simulink model "robot_capteur_etu"  (R2022a)
settings: Solver=VariableStepAuto  StartTime=0.0  StopTime=10.0  RelTol=1e-3
values from neighbouring files (symbols this model uses):
  K = -place(A,B,[-136.4009, -2.6408, -3.5890, -5.9800])    [matrices.m]    (also in simu_robot_etu.m = [0.6700 19.9055 1.0747  1.9614])
  ue = 0    [simu_robot_etu.m]
  x0 = [0 pi/10 0 0]    [simu_robot_etu.m]
  xe = [0 0 0 0]'    [simu_robot_etu.m]
settings Model: Creator=melallem  LastModifiedBy=elgue
settings DebuggingCC: UnconnectedInputMsg=warning  UnconnectedOutputMsg=warning  UnconnectedLineMsg=warning
settings RTWCC: DLArmComputeVersion=19.05

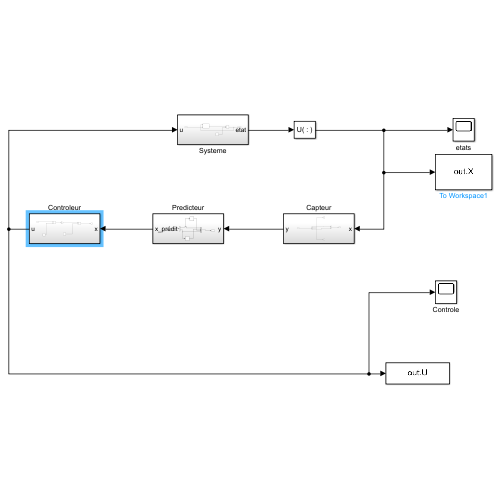
[thumbnail: Simulink's stored preview of the top-level diagram]
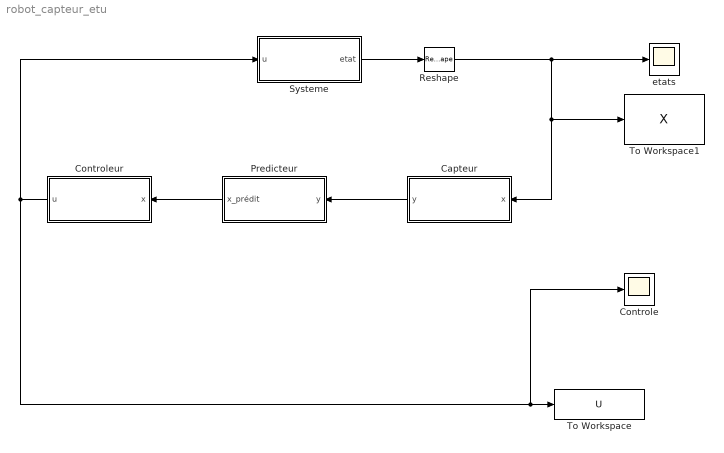
== system robot_capteur_etu ==
  Capteur : Subsystem
  Controle : Scope
  Controleur : Subsystem
  Predicteur : Subsystem
  Reshape : Reshape
  Systeme : Subsystem
  To Workspace : ToWorkspace  VariableName=U  SaveFormat=Timeseries  SampleTime=-1
  To Workspace1 : ToWorkspace  VariableName=X  SaveFormat=Timeseries  SampleTime=-1
  etats : Scope
  wires:
  Predicteur/1(x_prédit) -> Controleur/1(x)
  Capteur/1(y) -> Predicteur/1(y)
  Systeme/1(etat) -> Reshape/1
  Controleur/1(u) -> Controle/1, To Workspace/1, Systeme/1(u)
  Reshape/1 -> To Workspace1/1, Capteur/1(x), etats/1

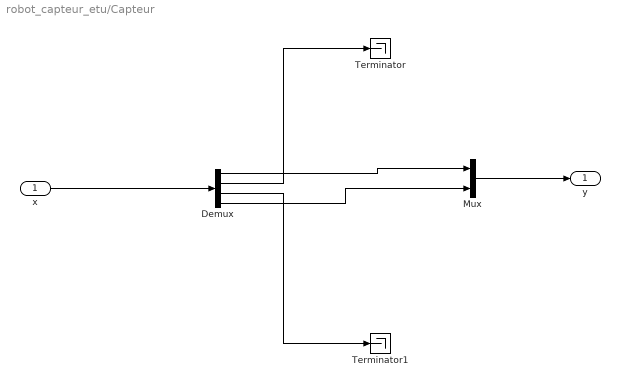
== system robot_capteur_etu/Capteur ==
  x : Inport
  Demux : Demux
  Mux : Mux  Inputs=2
  Terminator : Terminator
  Terminator1 : Terminator
  y : Outport
  wires:
  x/1 -> Demux/1
  Mux/1 -> y/1
  Demux/4 -> Mux/2
  Demux/3 -> Terminator1/1
  Demux/2 -> Terminator/1
  Demux/1 -> Mux/1

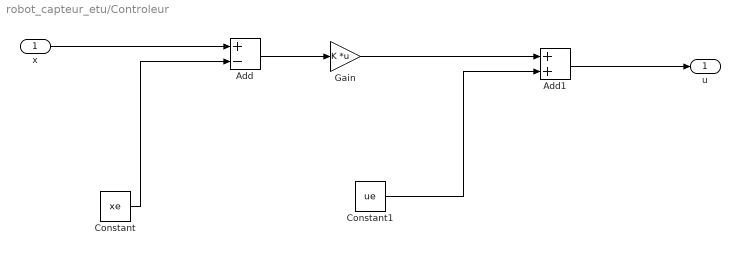
== system robot_capteur_etu/Controleur ==
  x : Inport
  Add : Sum  Inputs=+-
  Add1 : Sum
  Constant : Constant  Value=xe
  Constant1 : Constant  Value=ue
  Gain : Gain  Gain=K  Multiplication=Matrix(K*u)
  u : Outport
  wires:
  x/1 -> Add/1
  Constant/1 -> Add/2
  Add/1 -> Gain/1
  Gain/1 -> Add1/1
  Add1/1 -> u/1
  Constant1/1 -> Add1/2

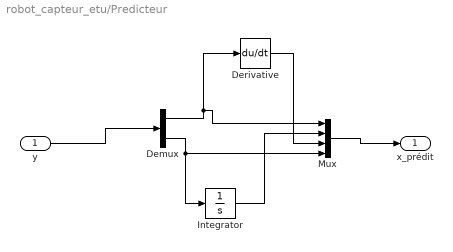
== system robot_capteur_etu/Predicteur ==
  y : Inport
  Demux : Demux  Outputs=2
  Derivative : Derivative
  Integrator : Integrator  InitialCondition=x0(2)
  Mux : Mux
  x_prédit : Outport
  wires:
  y/1 -> Demux/1
  Demux/1 -> Derivative/1, Mux/1
  Demux/2 -> Mux/4, Integrator/1
  Integrator/1 -> Mux/2
  Derivative/1 -> Mux/3
  Mux/1 -> x_prédit/1

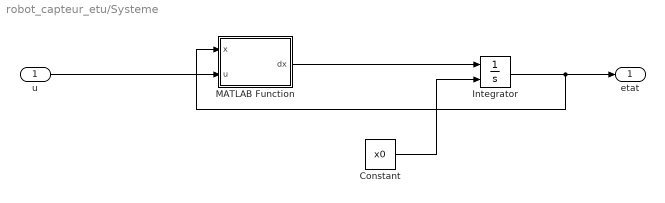
== system robot_capteur_etu/Systeme ==
  u : Inport
  Constant : Constant  Value=x0
  Integrator : Integrator  InitialConditionSource=external
  MATLAB Function : MATLAB Function  TreatAsAtomicUnit=on
  etat : Outport
  wires:
  u/1 -> MATLAB Function/2(u)
  Constant/1 -> Integrator/2
  MATLAB Function/1(dx) -> Integrator/1
  Integrator/1 -> etat/1, MATLAB Function/1(x)

== matlab function robot_capteur_etu/Systeme/MATLAB Function ==
  data: x input; u input; dx output
function dx = fcn(x,u)
dx = fonction(x,u);
